simulink model "pulse_detector_axis_zcu111"  (R2019b)
settings: Solver=FixedStepDiscrete  StartTime=0.0  StopTime=SimTime  RelTol=1e-3
PreLoadFcn:
  | model_init
InitFcn:
  | model_init
values from neighbouring files (symbols this model uses):
  CorrFilter = transpose(CorrFilter)    [model_init.m]
  RxSignal = RxSignal/scale1    [model_init.m]
  threshold = 0.03    [model_init.m]
  WindowLen = 11    [model_init.m]
libraries: hdlsllib x11, simulink x3, dspsrcs4 x2
Description:
  | DAC_ADC_DataCapture_TwoChan
  | 
  | RFSoC Data capture model that can stream two channels back over to DMA using a 128-bit data width
settings Model: DataTypeOverride=Off  Creator=mfornero  LastModifiedBy=tmealey
settings DataIOCC: SaveOutput=off  SaveTime=off  ReturnWorkspaceOutputs=off
settings OptimizationCC: BlockReduction=off  ConditionallyExecuteInputs=off  DefaultParameterBehavior=Inlined  LifeSpan=inf
settings DebuggingCC: AlgebraicLoopMsg=error  SingleTaskRateTransMsg=error  PregeneratedLibrarySubsystemCodeDiagnostic=none  StrictBusMsg=ErrorOnBusTreatedAsVector  SFUnexpectedBacktrackingDiag=warning  SFNoUnconditionalDefaultTransitionDiag=warning  SFExecutionAtInitializationDiag=none  ArithmeticOperatorsInVariantConditions=warning
settings HardwareCC: ProdBitPerPointer=32  ProdBitPerSizeT=32  ProdBitPerPtrDiffT=32  ProdLargestAtomicFloat=None  ProdIntDivRoundTo=Undefined  ProdEndianess=Unspecified  ProdWordSize=32  ProdHWDeviceType=ASIC/FPGA->ASIC/FPGA  ProdEqTarget=off
settings SFSimCC: SimUseLocalCustomCode=off  CustomCodeUndefinedFunction=UseInterfaceOnly
settings RTWCC: RTWUseLocalCustomCode=off
settings CodeAppCC: StateflowObjectComments=on
settings GRTTargetCC: TargetLangStandard=C89/C90 (ANSI)
settings ConfigComp: CovMetricSettings=dw  CovHtmlReporting=on  CovSaveCumulativeToWorkspaceVar=on  CovSaveSingleToWorkspaceVar=on  CovExternalEMLEnable=off

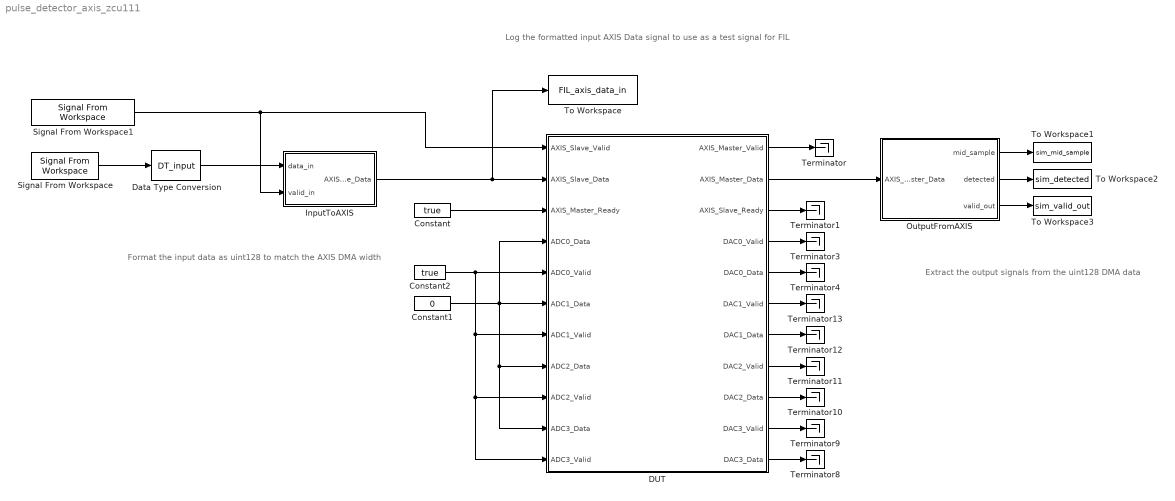
== system pulse_detector_axis_zcu111 ==
  note: Extract the output signals from the uint128 DMA data
  note: Format the input data as uint128 to match the AXIS DMA width
  note: Log the formatted input AXIS Data signal to use as a test signal for FIL
  Constant : Constant  Value=true  SampleTime=-1
  Constant1 : Constant  Value=0  OutDataTypeStr=fixdt(0,64,0)  SampleTime=-1
  Constant2 : Constant  Value=true  SampleTime=-1
  DUT : Subsystem  TreatAsAtomicUnit=on
  Data Type Conversion : DataTypeConversion  OutDataTypeStr=DT_input  RndMeth=Nearest  SaturateOnIntegerOverflow=on
  InputToAXIS : Subsystem
  OutputFromAXIS : Subsystem
  Signal From Workspace : dspsrcs4/Signal From Workspace  X=RxSignal  Ts=1  nsamps=1  OutputAfterFinalValue=Setting to zero  ignoreOrWarnInputAndFrameLengths=off  OutputFrames=off
  Signal From Workspace1 : dspsrcs4/Signal From Workspace  X=true(size(RxSignal))  Ts=1  nsamps=1  OutputAfterFinalValue=Setting to zero  ignoreOrWarnInputAndFrameLengths=off  OutputFrames=off
  Terminator{,1,3..4,8..13} (10 alike) : Terminator
  To Workspace : ToWorkspace  VariableName=FIL_axis_data_in  SampleTime=-1
      settings: Save2DSignal=2-D array (concatenate along first dimension)
  To Workspace1 : ToWorkspace  VariableName=sim_mid_sample  SampleTime=-1
      settings: Save2DSignal=2-D array (concatenate along first dimension)
  To Workspace2 : ToWorkspace  VariableName=sim_detected  SampleTime=-1
      settings: Save2DSignal=2-D array (concatenate along first dimension)
  To Workspace3 : ToWorkspace  VariableName=sim_valid_out  SampleTime=-1
      settings: Save2DSignal=2-D array (concatenate along first dimension)
  wires:
  Constant2/1 -> DUT/11("ADC3_Valid "), DUT/9(ADC2_Valid), DUT/7(ADC1_Valid), DUT/5(ADC0_Valid)
  Constant/1 -> DUT/3(AXIS_Master_Ready)
  DUT/3(AXIS_Slave_Ready) -> Terminator1/1
  DUT/6(DAC1_Valid) -> Terminator13/1
  DUT/7(DAC1_Data) -> Terminator12/1
  DUT/8(DAC2_Valid) -> Terminator11/1
  DUT/9(DAC2_Data) -> Terminator10/1
  DUT/10(DAC3_Valid) -> Terminator9/1
  DUT/11(DAC3_Data) -> Terminator8/1
  Constant1/1 -> DUT/10(ADC3_Data), DUT/8(ADC2_Data), DUT/4("ADC0_Data "), DUT/6(ADC1_Data)
  DUT/2(AXIS_Master_Data) -> OutputFromAXIS/1(AXIS_Master_Data)
  DUT/1(AXIS_Master_Valid) -> Terminator/1
  DUT/4(DAC0_Valid) -> Terminator3/1
  DUT/5(DAC0_Data) -> Terminator4/1
  Signal From Workspace1/1 -> InputToAXIS/2(valid_in), DUT/1(AXIS_Slave_Valid)
  Data Type Conversion/1 -> InputToAXIS/1(data_in)
  InputToAXIS/1(AXIS_Slave_Data) -> To Workspace/1, DUT/2(AXIS_Slave_Data)
  OutputFromAXIS/1(mid_sample) -> To Workspace1/1
  OutputFromAXIS/2(detected) -> To Workspace2/1
  OutputFromAXIS/3(valid_out) -> To Workspace3/1
  Signal From Workspace/1 -> Data Type Conversion/1

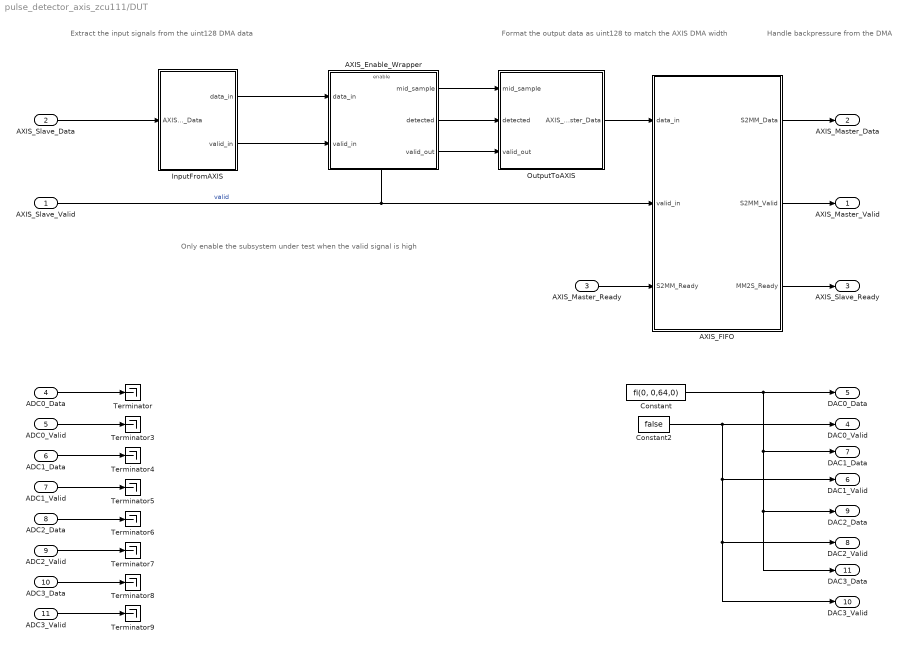
== system pulse_detector_axis_zcu111/DUT ==
  note: Handle backpressure from the DMA
  note: Only enable the subsystem under test when the valid signal is high
  note: Extract the input signals from the uint128 DMA data
  note: Format the output data as uint128 to match the AXIS DMA width
  AXIS_Slave_Valid : Inport
  AXIS_Slave_Data : Inport  Port=2
  AXIS_Master_Ready : Inport  Port=3
  "ADC0_Data " : Inport  Port=4
  ADC0_Valid : Inport  Port=5
  ADC1_Data : Inport  Port=6
  ADC1_Valid : Inport  Port=7
  ADC2_Data : Inport  Port=8
  ADC2_Valid : Inport  Port=9
  ADC3_Data : Inport  Port=10
  "ADC3_Valid " : Inport  Port=11
  AXIS_Enable_Wrapper : Subsystem
  AXIS_FIFO : Subsystem
  Constant : Constant  Value=fi(0, 0,64,0)  SampleTime=-1
  Constant2 : Constant  Value=false  OutDataTypeStr=boolean  SampleTime=-1
  InputFromAXIS : Subsystem
  OutputToAXIS : Subsystem
  Terminator{,3..9} (8 alike) : Terminator
  AXIS_Master_Valid : Outport  VectorParamsAs1DForOutWhenUnconnected=off
  AXIS_Master_Data : Outport  Port=2  VectorParamsAs1DForOutWhenUnconnected=off
  AXIS_Slave_Ready : Outport  Port=3  VectorParamsAs1DForOutWhenUnconnected=off
  DAC0_Valid : Outport  Port=4  VectorParamsAs1DForOutWhenUnconnected=off
  DAC0_Data : Outport  Port=5  VectorParamsAs1DForOutWhenUnconnected=off
  DAC1_Valid : Outport  Port=6  VectorParamsAs1DForOutWhenUnconnected=off
  DAC1_Data : Outport  Port=7  VectorParamsAs1DForOutWhenUnconnected=off
  DAC2_Valid : Outport  Port=8  VectorParamsAs1DForOutWhenUnconnected=off
  DAC2_Data : Outport  Port=9  VectorParamsAs1DForOutWhenUnconnected=off
  DAC3_Valid : Outport  Port=10  VectorParamsAs1DForOutWhenUnconnected=off
  DAC3_Data : Outport  Port=11  VectorParamsAs1DForOutWhenUnconnected=off
  wires:
  "ADC0_Data "/1 -> Terminator/1
  ADC0_Valid/1 -> Terminator3/1
  AXIS_Slave_Data/1 -> InputFromAXIS/1(AXIS_Slave_Data)
  AXIS_FIFO/3(MM2S_Ready) -> AXIS_Slave_Ready/1
  Constant2/1 -> DAC3_Valid/1, DAC2_Valid/1, DAC1_Valid/1, DAC0_Valid/1
  ADC1_Data/1 -> Terminator4/1
  ADC1_Valid/1 -> Terminator5/1
  ADC2_Data/1 -> Terminator6/1
  ADC2_Valid/1 -> Terminator7/1
  "ADC3_Valid "/1 -> Terminator9/1
  ADC3_Data/1 -> Terminator8/1
  Constant/1 -> DAC3_Data/1, DAC2_Data/1, DAC1_Data/1, DAC0_Data/1
  AXIS_Enable_Wrapper/1(mid_sample) -> OutputToAXIS/1(mid_sample)
  InputFromAXIS/2(valid_in) -> AXIS_Enable_Wrapper/2(valid_in)
  AXIS_Enable_Wrapper/3(valid_out) -> OutputToAXIS/3(valid_out)
  InputFromAXIS/1(data_in) -> AXIS_Enable_Wrapper/1(data_in)
  AXIS_Enable_Wrapper/2(detected) -> OutputToAXIS/2(detected)
  AXIS_Slave_Valid/1 -> AXIS_Enable_Wrapper/Enable, AXIS_FIFO/2(valid_in)  "valid"
  OutputToAXIS/1(AXIS_Master_Data) -> AXIS_FIFO/1(data_in)
  AXIS_FIFO/1(S2MM_Data) -> AXIS_Master_Data/1
  AXIS_Master_Ready/1 -> AXIS_FIFO/3(S2MM_Ready)
  AXIS_FIFO/2(S2MM_Valid) -> AXIS_Master_Valid/1

== system pulse_detector_axis_zcu111/InputToAXIS ==
  data_in : Inport
  valid_in : Inport  Port=2
  Bit Concat : hdlsllib/Logic and Bit Operations/Bit Concat  numInputs=4
      settings: SourceProductName=Simulink
  Complex to Real-Imag : ComplexToRealImag
  Constant : Constant  Value=0  OutDataTypeStr=fixdt(0,31+64,0)  SampleTime=-1
  AXIS_Slave_Data : Outport  VectorParamsAs1DForOutWhenUnconnected=off
  wires:
  Bit Concat/1 -> AXIS_Slave_Data/1
  data_in/1 -> Complex to Real-Imag/1
  valid_in/1 -> Bit Concat/4
  Complex to Real-Imag/1 -> Bit Concat/2
  Complex to Real-Imag/2 -> Bit Concat/3
  Constant/1 -> Bit Concat/1

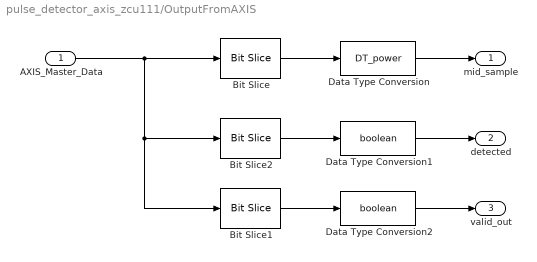
== system pulse_detector_axis_zcu111/OutputFromAXIS ==
  AXIS_Master_Data : Inport
  Bit Slice : hdlsllib/Logic and Bit Operations/Bit Slice  lidx=19  ridx=2
      settings: SourceProductName=Simulink  SourceProductBaseCode=SL
  Bit Slice1 : hdlsllib/Logic and Bit Operations/Bit Slice  lidx=0  ridx=0
      settings: SourceProductName=Simulink  SourceProductBaseCode=SL
  Bit Slice2 : hdlsllib/Logic and Bit Operations/Bit Slice  lidx=1  ridx=1
      settings: SourceProductName=Simulink  SourceProductBaseCode=SL
  Data Type Conversion : DataTypeConversion  OutDataTypeStr=DT_power  ConvertRealWorld=Stored Integer (SI)
  Data Type Conversion1 : DataTypeConversion  OutDataTypeStr=boolean
  Data Type Conversion2 : DataTypeConversion  OutDataTypeStr=boolean
  mid_sample : Outport  VectorParamsAs1DForOutWhenUnconnected=off
  detected : Outport  Port=2  VectorParamsAs1DForOutWhenUnconnected=off
  valid_out : Outport  Port=3  VectorParamsAs1DForOutWhenUnconnected=off
  wires:
  AXIS_Master_Data/1 -> Bit Slice1/1, Bit Slice2/1, Bit Slice/1
  Bit Slice/1 -> Data Type Conversion/1
  Data Type Conversion/1 -> mid_sample/1
  Bit Slice2/1 -> Data Type Conversion1/1
  Data Type Conversion1/1 -> detected/1
  Data Type Conversion2/1 -> valid_out/1
  Bit Slice1/1 -> Data Type Conversion2/1

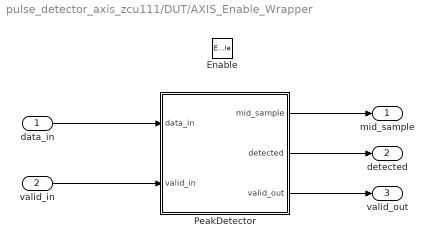
== system pulse_detector_axis_zcu111/DUT/AXIS_Enable_Wrapper ==
  data_in : Inport
  valid_in : Inport  Port=2
  Enable : EnablePort
  PeakDetector : Subsystem
  mid_sample : Outport  InitialOutput=0  VectorParamsAs1DForOutWhenUnconnected=off
  detected : Outport  Port=2  InitialOutput=0  VectorParamsAs1DForOutWhenUnconnected=off
  valid_out : Outport  Port=3  InitialOutput=0  VectorParamsAs1DForOutWhenUnconnected=off
  wires:
  data_in/1 -> PeakDetector/1(data_in)
  valid_in/1 -> PeakDetector/2(valid_in)
  PeakDetector/1(mid_sample) -> mid_sample/1
  PeakDetector/2(detected) -> detected/1
  PeakDetector/3(valid_out) -> valid_out/1

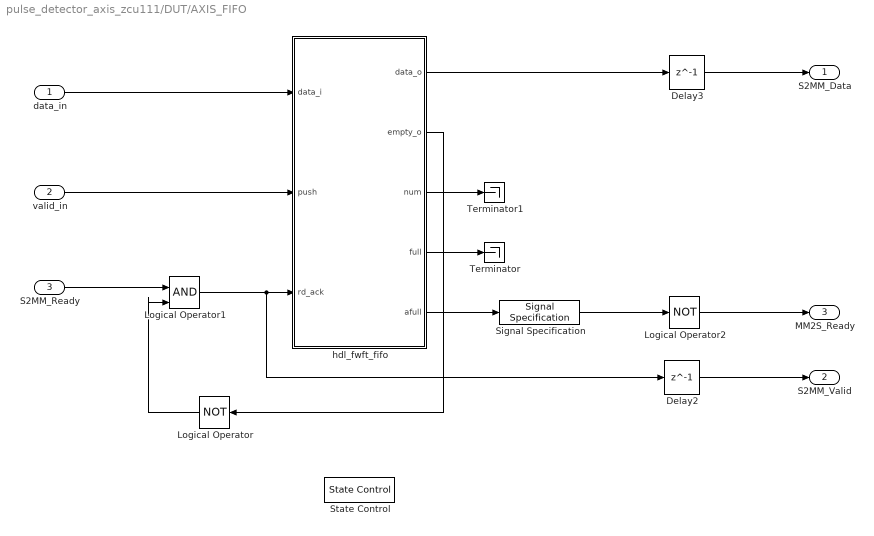
== system pulse_detector_axis_zcu111/DUT/AXIS_FIFO ==
  data_in : Inport
  valid_in : Inport  Port=2
  S2MM_Ready : Inport  Port=3
  Delay2 : Delay  DelayLength=1
  Delay3 : Delay  DelayLength=1
  Logical Operator : Logic  Operator=NOT  IconShape=distinctive  AllPortsSameDT=off  OutDataTypeStr=boolean
  Logical Operator1 : Logic  IconShape=distinctive  AllPortsSameDT=off  OutDataTypeStr=boolean
  Logical Operator2 : Logic  Operator=NOT  IconShape=distinctive  AllPortsSameDT=off  OutDataTypeStr=boolean
  Signal Specification : SignalSpecification  Dimensions=1  SampleTime=1
  State Control : StateControl  StateControl=Synchronous
  Terminator : Terminator
  Terminator1 : Terminator
  hdl_fwft_fifo : Subsystem  mask{FIFO_DEPTH=16, AFULL_THRESH=8}
      mask prompts: FIFO_DEPTH "FIFO Depth"; AFULL_THRESH "Almost Full Threshold"
      mask init:
      | FIFO_CNT_BITS=ceil(log2(FIFO_DEPTH+1+3));
  S2MM_Data : Outport  VectorParamsAs1DForOutWhenUnconnected=off
  S2MM_Valid : Outport  Port=2  VectorParamsAs1DForOutWhenUnconnected=off
  MM2S_Ready : Outport  Port=3  VectorParamsAs1DForOutWhenUnconnected=off
  wires:
  Signal Specification/1 -> Logical Operator2/1
  hdl_fwft_fifo/5(afull) -> Signal Specification/1
  hdl_fwft_fifo/2(empty_o) -> Logical Operator/1
  Logical Operator2/1 -> MM2S_Ready/1
  hdl_fwft_fifo/3(num) -> Terminator1/1
  hdl_fwft_fifo/4(full) -> Terminator/1
  Logical Operator/1 -> Logical Operator1/2
  S2MM_Ready/1 -> Logical Operator1/1
  Logical Operator1/1 -> Delay2/1, hdl_fwft_fifo/3(rd_ack)
  Delay2/1 -> S2MM_Valid/1
  valid_in/1 -> hdl_fwft_fifo/2(push)
  Delay3/1 -> S2MM_Data/1
  hdl_fwft_fifo/1(data_o) -> Delay3/1
  data_in/1 -> hdl_fwft_fifo/1(data_i)

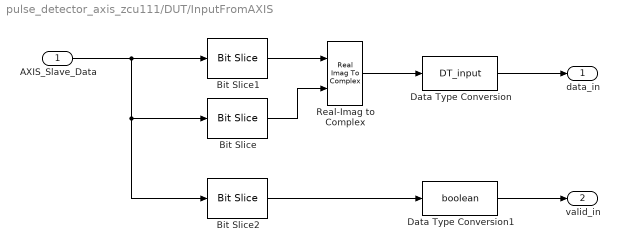
== system pulse_detector_axis_zcu111/DUT/InputFromAXIS ==
  AXIS_Slave_Data : Inport
  Bit Slice : hdlsllib/Logic and Bit Operations/Bit Slice  lidx=16  ridx=1
      settings: SourceProductName=Simulink  SourceProductBaseCode=SL
  Bit Slice1 : hdlsllib/Logic and Bit Operations/Bit Slice  lidx=32  ridx=17
      settings: SourceProductName=Simulink  SourceProductBaseCode=SL
  Bit Slice2 : hdlsllib/Logic and Bit Operations/Bit Slice  lidx=0  ridx=0
      settings: SourceProductName=Simulink  SourceProductBaseCode=SL
  Data Type Conversion : DataTypeConversion  OutDataTypeStr=DT_input  ConvertRealWorld=Stored Integer (SI)
  Data Type Conversion1 : DataTypeConversion  OutDataTypeStr=boolean
  Real-Imag to Complex : RealImagToComplex
  data_in : Outport  VectorParamsAs1DForOutWhenUnconnected=off
  valid_in : Outport  Port=2  VectorParamsAs1DForOutWhenUnconnected=off
  wires:
  AXIS_Slave_Data/1 -> Bit Slice2/1, Bit Slice/1, Bit Slice1/1
  Data Type Conversion/1 -> data_in/1
  Bit Slice2/1 -> Data Type Conversion1/1
  Data Type Conversion1/1 -> valid_in/1
  Bit Slice1/1 -> Real-Imag to Complex/1
  Bit Slice/1 -> Real-Imag to Complex/2
  Real-Imag to Complex/1 -> Data Type Conversion/1

== system pulse_detector_axis_zcu111/DUT/OutputToAXIS ==
  mid_sample : Inport
  detected : Inport  Port=2
  valid_out : Inport  Port=3
  Bit Concat : hdlsllib/Logic and Bit Operations/Bit Concat  numInputs=4
      settings: SourceProductName=Simulink
  Constant : Constant  Value=0  OutDataTypeStr=fixdt(0,108,0)  SampleTime=-1
  AXIS_Master_Data : Outport  VectorParamsAs1DForOutWhenUnconnected=off
  wires:
  Bit Concat/1 -> AXIS_Master_Data/1
  Constant/1 -> Bit Concat/1
  mid_sample/1 -> Bit Concat/2
  detected/1 -> Bit Concat/3
  valid_out/1 -> Bit Concat/4

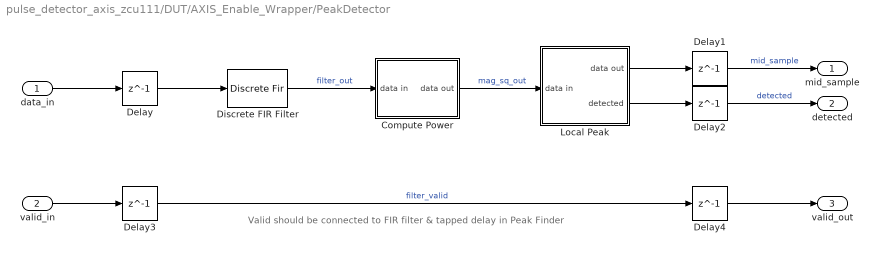
== system pulse_detector_axis_zcu111/DUT/AXIS_Enable_Wrapper/PeakDetector ==
  note: Valid should be connected to FIR filter & tapped delay in Peak Finder
  data_in : Inport  OutDataTypeStr=DT_input
      settings: SignalType=complex
  valid_in : Inport  Port=2  OutDataTypeStr=boolean
  Compute Power : Subsystem
      settings: AttributesFormatString=|
      | Architecture : Module
      | AdaptivePipelining : on
      | InputPipeline : 1
      | OutputPipeline : 1
  Delay{,1..4} (5 alike) : Delay  DelayLength=1
  Discrete FIR Filter : DiscreteFir  FilterStructure=Direct form transposed  Coefficients=CorrFilter  CoefDataTypeStr=DT_coeff
      settings: AttributesFormatString=|
      | Architecture : Fully Parallel
      | InputPipeline : 1
      | MultiplierInputPipeline : 1
      | MultiplierOutputPipeline : 1
      | OutputPipeline : 1
  Local Peak : Subsystem
  mid_sample : Outport  VectorParamsAs1DForOutWhenUnconnected=off
  detected : Outport  Port=2  VectorParamsAs1DForOutWhenUnconnected=off
  valid_out : Outport  Port=3  VectorParamsAs1DForOutWhenUnconnected=off
  wires:
  Discrete FIR Filter/1 -> Compute Power/1(data in)  "filter_out"
  Local Peak/1(data out) -> Delay1/1
  Compute Power/1(data out) -> Local Peak/1(data in)  "mag_sq_out"
  Delay4/1 -> valid_out/1
  Delay3/1 -> Delay4/1  "filter_valid"
  valid_in/1 -> Delay3/1
  Local Peak/2(detected) -> Delay2/1
  Delay1/1 -> mid_sample/1  "mid_sample"
  Delay/1 -> Discrete FIR Filter/1
  data_in/1 -> Delay/1
  Delay2/1 -> detected/1  "detected"

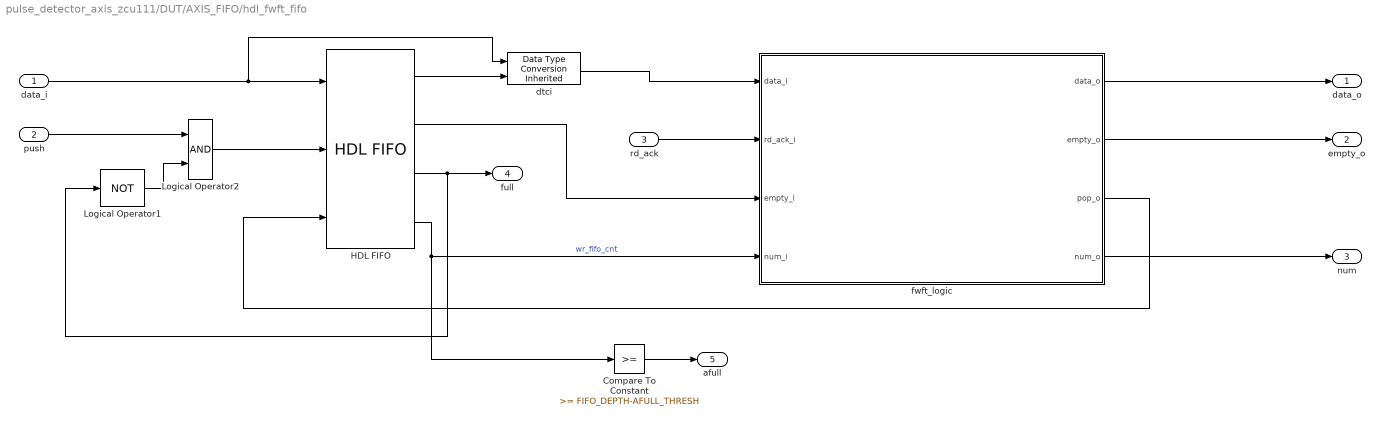
== system pulse_detector_axis_zcu111/DUT/AXIS_FIFO/hdl_fwft_fifo ==
  data_i : Inport
  push : Inport  Port=2
  rd_ack : Inport  Port=3
  Compare To Constant : simulink/Logic and Bit Operations/Compare To Constant  relop=>=  const=FIFO_DEPTH-AFULL_THRESH  OutDataTypeStr=boolean
  HDL FIFO : hdlsllib/HDL RAMs/HDL FIFO  fifo_size=FIFO_DEPTH  mode=Classic  ratio=1  push_msg=Error  pop_msg=Ignore  show_empty=on  show_full=on  show_num=on  LabelModeActiveChoice_Mode=Classic
      settings: SourceProductName=HDL Coder  SourceProductBaseCode=HD
  Logical Operator1 : Logic  Operator=NOT  IconShape=distinctive  AllPortsSameDT=off  OutDataTypeStr=boolean
  Logical Operator2 : Logic  IconShape=distinctive  AllPortsSameDT=off  OutDataTypeStr=boolean
  dtci : simulink/Signal Attributes/Data Type Conversion Inherited  ConvertRealWorld=Real World Value  DoSatur=off
      settings: SourceProductName=Simulink  SourceProductBaseCode=SL
  fwft_logic : Subsystem
  data_o : Outport  VectorParamsAs1DForOutWhenUnconnected=off
  empty_o : Outport  Port=2  VectorParamsAs1DForOutWhenUnconnected=off
  num : Outport  Port=3  VectorParamsAs1DForOutWhenUnconnected=off
  full : Outport  Port=4  VectorParamsAs1DForOutWhenUnconnected=off
  afull : Outport  Port=5  VectorParamsAs1DForOutWhenUnconnected=off
  wires:
  fwft_logic/4(num_o) -> num/1
  HDL FIFO/4 -> fwft_logic/4(num_i), Compare To Constant/1  "wr_fifo_cnt"
  HDL FIFO/3 -> full/1, Logical Operator1/1
  dtci/1 -> fwft_logic/1(data_i)
  HDL FIFO/1 -> dtci/2
  Logical Operator1/1 -> Logical Operator2/2
  Logical Operator2/1 -> HDL FIFO/2
  push/1 -> Logical Operator2/1
  fwft_logic/3(pop_o) -> HDL FIFO/3
  data_i/1 -> HDL FIFO/1, dtci/1
  fwft_logic/2(empty_o) -> empty_o/1
  rd_ack/1 -> fwft_logic/2(rd_ack_i)
  HDL FIFO/2 -> fwft_logic/3(empty_i)
  fwft_logic/1(data_o) -> data_o/1
  Compare To Constant/1 -> afull/1

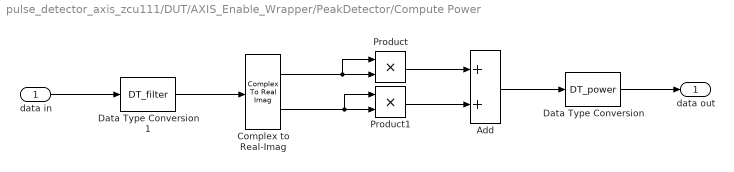
== system pulse_detector_axis_zcu111/DUT/AXIS_Enable_Wrapper/PeakDetector/Compute Power ==
  data in : Inport
  Add : Sum
  Complex to Real-Imag : ComplexToRealImag
  Data Type Conversion : DataTypeConversion  OutDataTypeStr=DT_power
  Data Type Conversion1 : DataTypeConversion  OutDataTypeStr=DT_filter
  Product : Product
  Product1 : Product
  data out : Outport  VectorParamsAs1DForOutWhenUnconnected=off
  wires:
  Complex to Real-Imag/1 -> Product/1, Product/2
  Complex to Real-Imag/2 -> Product1/1, Product1/2
  Product1/1 -> Add/2
  Product/1 -> Add/1
  data in/1 -> Data Type Conversion1/1
  Add/1 -> Data Type Conversion/1
  Data Type Conversion/1 -> data out/1
  Data Type Conversion1/1 -> Complex to Real-Imag/1

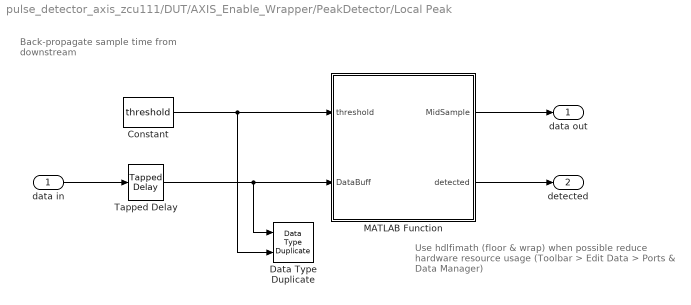
== system pulse_detector_axis_zcu111/DUT/AXIS_Enable_Wrapper/PeakDetector/Local Peak ==
  note: Use hdlfimath (floor & wrap) when possible
      | reduce hardware resource usage
      | (Toolbar > Edit Data > Ports & Data Manager)
  note: Back-propagate sample time
      | from downstream
  data in : Inport
  Constant : Constant  Value=threshold  OutDataTypeStr=Inherit: Inherit via back propagation  SampleTime=-1
  Data Type Duplicate : DataTypeDuplicate
  MATLAB Function : MATLAB Function  TreatAsAtomicUnit=on
  Tapped Delay : simulink/Discrete/Tapped Delay  vinit=0.0  samptime=-1  NumDelays=WindowLen  DelayOrder=Oldest  includeCurrent=off
  data out : Outport  VectorParamsAs1DForOutWhenUnconnected=off
  detected : Outport  Port=2  VectorParamsAs1DForOutWhenUnconnected=off
  wires:
  data in/1 -> Tapped Delay/1
  Constant/1 -> Data Type Duplicate/2, MATLAB Function/1(threshold)
  MATLAB Function/1(MidSample) -> data out/1
  MATLAB Function/2(detected) -> detected/1
  Tapped Delay/1 -> Data Type Duplicate/1, MATLAB Function/2(DataBuff)

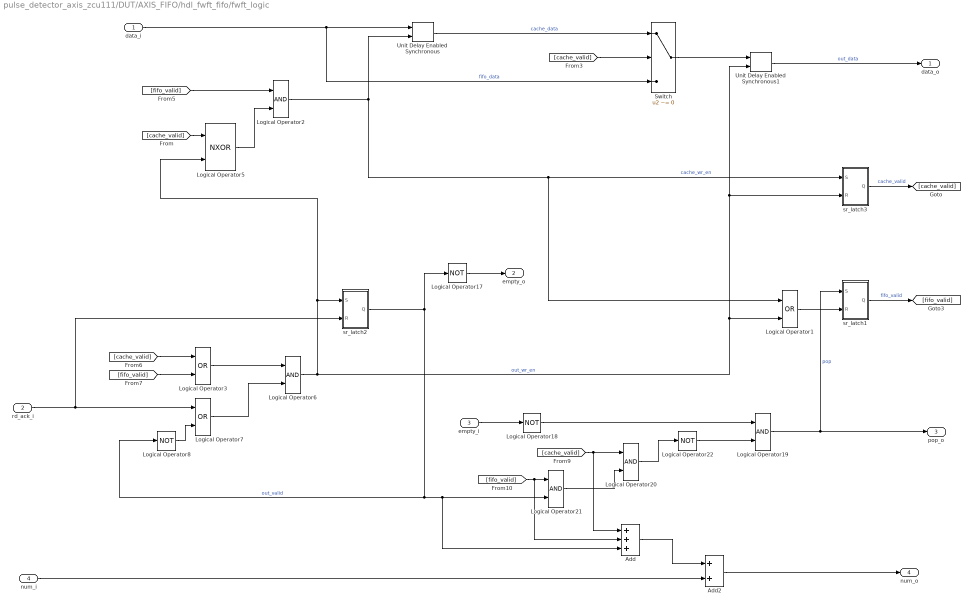
== system pulse_detector_axis_zcu111/DUT/AXIS_FIFO/hdl_fwft_fifo/fwft_logic ==
  data_i : Inport
  rd_ack_i : Inport  Port=2
  empty_i : Inport  Port=3
  num_i : Inport  Port=4
  Add : Sum  Inputs=+++  AccumDataTypeStr=fixdt(0,2,0)
  Add2 : Sum  OutDataTypeStr=fixdt(0,FIFO_CNT_BITS,0)
  Logical Operator1 : Logic  Operator=OR  IconShape=distinctive  AllPortsSameDT=off  OutDataTypeStr=boolean
  Logical Operator{8,17..18,22} (4 alike) : Logic  Operator=NOT  IconShape=distinctive  AllPortsSameDT=off  OutDataTypeStr=boolean
  Logical Operator{2,6,19..21} (5 alike) : Logic  IconShape=distinctive  AllPortsSameDT=off  OutDataTypeStr=boolean
  Logical Operator3 : Logic  Operator=OR  IconShape=distinctive  AllPortsSameDT=off  OutDataTypeStr=boolean
  Logical Operator5 : Logic  Operator=NXOR  IconShape=distinctive  AllPortsSameDT=off  OutDataTypeStr=boolean
  Logical Operator7 : Logic  Operator=OR  IconShape=distinctive  AllPortsSameDT=off  OutDataTypeStr=boolean
  Switch : Switch  Criteria=u2 ~= 0
  Unit Delay Enabled Synchronous : hdlsllib/Discrete/Unit Delay Enabled Synchronous  InitialCondition=0.0  SampleTime=-1
      settings: SourceProductName=Simulink  SourceProductBaseCode=SL
  Unit Delay Enabled Synchronous1 : hdlsllib/Discrete/Unit Delay Enabled Synchronous  InitialCondition=0.0  SampleTime=-1
      settings: SourceProductName=Simulink  SourceProductBaseCode=SL
  sr_latch1 : Subsystem
  sr_latch2 : Subsystem
  sr_latch3 : Subsystem
  data_o : Outport  VectorParamsAs1DForOutWhenUnconnected=off
  empty_o : Outport  Port=2  VectorParamsAs1DForOutWhenUnconnected=off
  pop_o : Outport  Port=3  VectorParamsAs1DForOutWhenUnconnected=off
  num_o : Outport  Port=4  VectorParamsAs1DForOutWhenUnconnected=off
  wires:
  Add2/1 -> num_o/1
  Add/1 -> Add2/1
  num_i/1 -> Add2/2
  Unit Delay Enabled Synchronous1/1 -> data_o/1  "out_data"
  Logical Operator1/1 -> sr_latch1/2(R)
  [fifo_valid] -> Logical Operator21/1, Add/2
  [cache_valid] -> Logical Operator20/1, Add/1
  Logical Operator19/1 -> pop_o/1, sr_latch1/1(S)  "pop"
  Logical Operator20/1 -> Logical Operator22/1
  Logical Operator22/1 -> Logical Operator19/2
  Logical Operator21/1 -> Logical Operator20/2
  Logical Operator18/1 -> Logical Operator19/1
  Logical Operator17/1 -> empty_o/1
  Logical Operator8/1 -> Logical Operator7/2
  sr_latch2/1(Q) -> Logical Operator17/1, Logical Operator21/2, Add/3, Logical Operator8/1  "out_valid"
  rd_ack_i/1 -> Logical Operator7/1, sr_latch2/2(R)
  Logical Operator7/1 -> Logical Operator6/2
  Logical Operator3/1 -> Logical Operator6/1
  [fifo_valid] -> Logical Operator3/2
  [cache_valid] -> Logical Operator3/1
  [fifo_valid] -> Logical Operator2/1
  Logical Operator2/1 -> Unit Delay Enabled Synchronous/2, Logical Operator1/1, sr_latch3/1(S)  "cache_wr_en"
  [cache_valid] -> Switch/2
  [cache_valid] -> Logical Operator5/1
  Logical Operator6/1 -> Logical Operator1/2, Unit Delay Enabled Synchronous1/2, sr_latch3/2(R), sr_latch2/1(S), Logical Operator5/2  "out_wr_en"
  Logical Operator5/1 -> Logical Operator2/2
  Unit Delay Enabled Synchronous/1 -> Switch/1  "cache_data"
  data_i/1 -> Unit Delay Enabled Synchronous/1, Switch/3  "fifo_data"
  Switch/1 -> Unit Delay Enabled Synchronous1/1
  sr_latch3/1(Q) -> [cache_valid]  "cache_valid"
  sr_latch1/1(Q) -> [fifo_valid]  "fifo_valid"
  empty_i/1 -> Logical Operator18/1

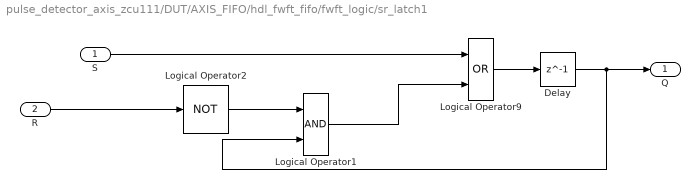
== system pulse_detector_axis_zcu111/DUT/AXIS_FIFO/hdl_fwft_fifo/fwft_logic/sr_latch1 ==
  S : Inport
  R : Inport  Port=2
  Delay : Delay  DelayLength=1
  Logical Operator1 : Logic  IconShape=distinctive  AllPortsSameDT=off  OutDataTypeStr=boolean
  Logical Operator2 : Logic  Operator=NOT  IconShape=distinctive  AllPortsSameDT=off  OutDataTypeStr=boolean
  Logical Operator9 : Logic  Operator=OR  IconShape=distinctive  AllPortsSameDT=off  OutDataTypeStr=boolean
  Q : Outport  VectorParamsAs1DForOutWhenUnconnected=off
  wires:
  S/1 -> Logical Operator9/1
  R/1 -> Logical Operator2/1
  Logical Operator2/1 -> Logical Operator1/1
  Delay/1 -> Logical Operator1/2, Q/1
  Logical Operator9/1 -> Delay/1
  Logical Operator1/1 -> Logical Operator9/2

== system pulse_detector_axis_zcu111/DUT/AXIS_FIFO/hdl_fwft_fifo/fwft_logic/sr_latch2 ==
  S : Inport
  R : Inport  Port=2
  Delay : Delay  DelayLength=1
  Logical Operator1 : Logic  IconShape=distinctive  AllPortsSameDT=off  OutDataTypeStr=boolean
  Logical Operator2 : Logic  Operator=NOT  IconShape=distinctive  AllPortsSameDT=off  OutDataTypeStr=boolean
  Logical Operator9 : Logic  Operator=OR  IconShape=distinctive  AllPortsSameDT=off  OutDataTypeStr=boolean
  Q : Outport  VectorParamsAs1DForOutWhenUnconnected=off
  wires:
  Logical Operator1/1 -> Logical Operator9/2
  Logical Operator9/1 -> Delay/1
  Delay/1 -> Q/1, Logical Operator1/2
  Logical Operator2/1 -> Logical Operator1/1
  R/1 -> Logical Operator2/1
  S/1 -> Logical Operator9/1

== system pulse_detector_axis_zcu111/DUT/AXIS_FIFO/hdl_fwft_fifo/fwft_logic/sr_latch3 ==
  S : Inport
  R : Inport  Port=2
  Delay : Delay  DelayLength=1
  Logical Operator1 : Logic  IconShape=distinctive  AllPortsSameDT=off  OutDataTypeStr=boolean
  Logical Operator2 : Logic  Operator=NOT  IconShape=distinctive  AllPortsSameDT=off  OutDataTypeStr=boolean
  Logical Operator9 : Logic  Operator=OR  IconShape=distinctive  AllPortsSameDT=off  OutDataTypeStr=boolean
  Q : Outport  VectorParamsAs1DForOutWhenUnconnected=off
  wires:
  Logical Operator1/1 -> Logical Operator9/2
  Logical Operator9/1 -> Delay/1
  Delay/1 -> Q/1, Logical Operator1/2
  Logical Operator2/1 -> Logical Operator1/1
  R/1 -> Logical Operator2/1
  S/1 -> Logical Operator9/1

== matlab function pulse_detector_axis_zcu111/DUT/AXIS_Enable_Wrapper/PeakDetector/Local Peak/MATLAB Function ==
  data: WindowLen parameter; threshold input; DataBuff input; MidSample output; detected output
function [MidSample,detected] = fcn(WindowLen, threshold, DataBuff)
%#codegen

% Hardware friendly implementation of peak finder
% Modify MATLAB reference as followed:
%
% Define function inputs:
% - WindowLen: non-tunable parameter defined under Simulink->Edit Data
% - threhold: input port (connected to constant)
% - DataBuff: input port (buffering done using Simulink block)
% Define function outputs:
% - Set "detected" when MidSample is local max

MidIdx = ceil(WindowLen/2);

% Compare each value in the window to the middle sample via subtraction
MidSample = DataBuff(MidIdx);
CompareOut = DataBuff - MidSample; % this is a vector

% if all values in the result are negative and the middle sample is
% greater than a threshold, it is a local max
if all(CompareOut <= 0) && (MidSample > threshold)
    detected = true;
else
    detected = false;
end
